simulink model "DSBSC"  (R2023b)
settings: Solver=VariableStepAuto  StartTime=0.0  StopTime=100  RelTol=1e-3
libraries: simulink x3, dspfdesign x1
settings Model: Creator=HP  LastModifiedBy=HP

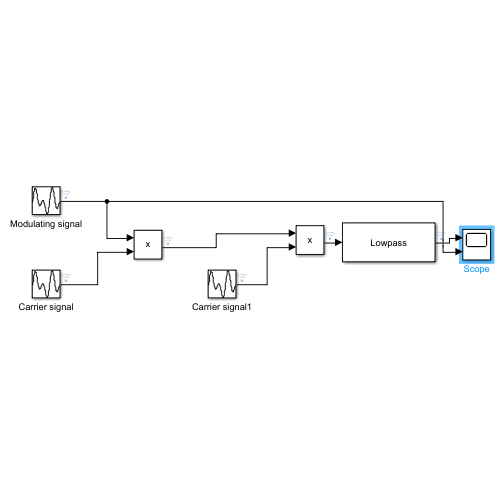
[thumbnail: Simulink's stored preview of the top-level diagram]
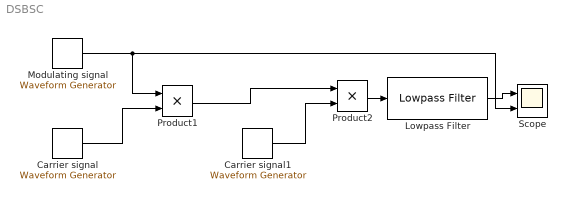
== system DSBSC ==
  Carrier signal : simulink/Sources/Waveform Generator  OutMin=[]  OutMax=[]  OutDataTypeStr=Inherit: Inherit via back propagation  SelectedSignal=1  Signals=sin(2,20,1)  BlockNames=MultiportSwitch_14b974e83f6d4c0  SampleTime=0.1
  Carrier signal1 : simulink/Sources/Waveform Generator  OutMin=[]  OutMax=[]  OutDataTypeStr=Inherit: Inherit via back propagation  SelectedSignal=1  Signals=sin(2,20,1)  BlockNames=MultiportSwitch_14b974e83f6d4c0  SampleTime=0.1
  Lowpass Filter : dspfdesign/Lowpass Filter  FilterType=FIR  DesignForMinimumOrder=on  FilterOrder=50  PassbandFrequency=8e3  StopbandFrequency=12e3  PassbandRipple=0.1  StopbandAttenuation=80  SampleRateMode=Specify on dialog  SampleRate=44100  SimulateUsing=Interpreted execution  roundingMode=Floor  coeffsDataTypeStr=fixdt(1,16)
  Modulating signal : simulink/Sources/Waveform Generator  OutMin=[]  OutMax=[]  OutDataTypeStr=Inherit: Inherit via back propagation  SelectedSignal=1  Signals=sin(5,5,1)  BlockNames=MultiportSwitch_1e26bf96150c493  SampleTime=0.1
  Product1 : Product
  Product2 : Product
  Scope : Scope  NumInputPorts=2
  wires:
  Carrier signal/1 -> Product1/2
  Product1/1 -> Product2/1
  Modulating signal/1 -> Scope/2, Product1/1
  Product2/1 -> Lowpass Filter/1
  Lowpass Filter/1 -> Scope/1
  Carrier signal1/1 -> Product2/2
